simulink model "TelescopeModel"  (R2016a)
settings: Solver=ode45  StartTime=0.0  StopTime=inf  RelTol=1e-3
libraries: simulink x2, vrlib x1
settings Model: Creator=Baris  LastModifiedBy=ds
settings DataIOCC: LimitDataPoints=on  SaveFormat=Array
settings DebuggingCC: SolverPrmCheckMsg=warning  AllowSymbolicDim=off
settings HardwareCC: ProdBitPerPointer=32  ProdLargestAtomicFloat=None  ProdIntDivRoundTo=Undefined  ProdEndianess=Unspecified  ProdWordSize=32  ProdHWDeviceType=32-bit Generic
settings ModelReferenceCC: PropagateSignalLabelsOutOfModel=off
settings ConfigComp: CovModelRefEnable=Off  CovSFcnEnable=off

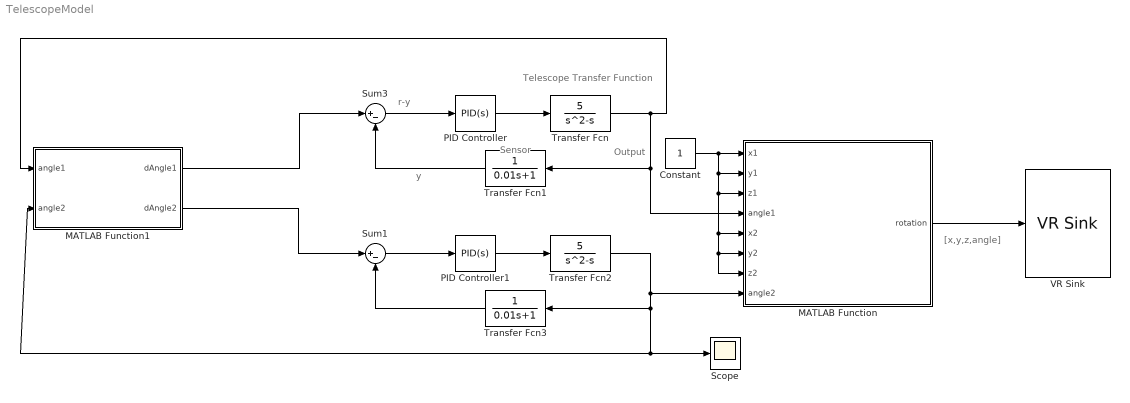
== system TelescopeModel ==
  note: [x,y,z,angle]
  note: r-y
  note: y
  note: Output
  note: Sensor
  note: Telescope Transfer Function
  Constant : Constant
  MATLAB Function : MATLAB Function  TreatAsAtomicUnit=on
  MATLAB Function1 : MATLAB Function  TreatAsAtomicUnit=on
  PID Controller : simulink/Continuous/PID Controller  Controller=PID  TimeDomain=Continuous-time  SampleTime=-1  IntegratorMethod=Forward Euler  FilterMethod=Forward Euler  Form=Ideal  UseFilter=on  ControllerParametersSource=internal  P=9.91044376883815  I=0.179707343353955  D=0.466765758106248  N=123.439816106141  InitialConditionSource=internal  InitialConditionForIntegrator=0  InitialConditionForFilter=0  ExternalReset=none  LimitOutput=off  UpperSaturationLimit=inf  LowerSaturationLimit=-inf  LinearizeAsGain=on  AntiWindupMode=none  Kb=1  TrackingMode=off  Kt=1  PParamMin=[]  PParamMax=[]  IParamMin=[]  IParamMax=[]  DParamMin=[]  DParamMax=[]  NParamMin=[]  NParamMax=[]  KbParamMin=[]  KbParamMax=[]  KtParamMin=[]  KtParamMax=[]  POutMin=[]  POutMax=[]  IOutMin=[]  IOutMax=[]  DOutMin=[]  DOutMax=[]  NOutMin=[]  NOutMax=[]  KbOutMin=[]  KbOutMax=[]  KtOutMin=[]  KtOutMax=[]  IntegratorOutMin=[]  IntegratorOutMax=[]  FilterOutMin=[]  FilterOutMax=[]  SumOutMin=[]  SumOutMax=[]  SumI1OutMin=[]  SumI1OutMax=[]  SumI2OutMin=[]  SumI2OutMax=[]  SumI3OutMin=[]  SumI3OutMax=[]  SumDOutMin=[]  SumDOutMax=[]  SaturationOutMin=[]  SaturationOutMax=[]  IntegratorContinuousStateAttributes=''  IntegratorStateMustResolveToSignalObject=off  IntegratorRTWStateStorageClass=Auto  FilterContinuousStateAttributes=''  FilterStateMustResolveToSignalObject=off  FilterRTWStateStorageClass=Auto  DifferentiatorICPrevScaledInput=0  DifferentiatorOutMin=[]  DifferentiatorOutMax=[]
  PID Controller1 : simulink/Continuous/PID Controller  Controller=PID  TimeDomain=Continuous-time  SampleTime=-1  IntegratorMethod=Forward Euler  FilterMethod=Forward Euler  Form=Ideal  UseFilter=on  ControllerParametersSource=internal  P=9.91044376883815  I=0.179707343353955  D=0.466765758106248  N=123.439816106141  InitialConditionSource=internal  InitialConditionForIntegrator=0  InitialConditionForFilter=0  ExternalReset=none  LimitOutput=off  UpperSaturationLimit=inf  LowerSaturationLimit=-inf  LinearizeAsGain=on  AntiWindupMode=none  Kb=1  TrackingMode=off  Kt=1  PParamMin=[]  PParamMax=[]  IParamMin=[]  IParamMax=[]  DParamMin=[]  DParamMax=[]  NParamMin=[]  NParamMax=[]  KbParamMin=[]  KbParamMax=[]  KtParamMin=[]  KtParamMax=[]  POutMin=[]  POutMax=[]  IOutMin=[]  IOutMax=[]  DOutMin=[]  DOutMax=[]  NOutMin=[]  NOutMax=[]  KbOutMin=[]  KbOutMax=[]  KtOutMin=[]  KtOutMax=[]  IntegratorOutMin=[]  IntegratorOutMax=[]  FilterOutMin=[]  FilterOutMax=[]  SumOutMin=[]  SumOutMax=[]  SumI1OutMin=[]  SumI1OutMax=[]  SumI2OutMin=[]  SumI2OutMax=[]  SumI3OutMin=[]  SumI3OutMax=[]  SumDOutMin=[]  SumDOutMax=[]  SaturationOutMin=[]  SaturationOutMax=[]  IntegratorContinuousStateAttributes=''  IntegratorStateMustResolveToSignalObject=off  IntegratorRTWStateStorageClass=Auto  FilterContinuousStateAttributes=''  FilterStateMustResolveToSignalObject=off  FilterRTWStateStorageClass=Auto  DifferentiatorICPrevScaledInput=0  DifferentiatorOutMin=[]  DifferentiatorOutMax=[]
  Scope : Scope
  Sum1 : Sum  Inputs=|+-
  Sum3 : Sum  Inputs=|+-
  Transfer Fcn : TransferFcn  Numerator=[5]  Denominator=[1 -1 0]
  Transfer Fcn1 : TransferFcn  Denominator=[0.01 1]
  Transfer Fcn2 : TransferFcn  Numerator=[5]  Denominator=[1 -1 0]
  Transfer Fcn3 : TransferFcn  Denominator=[0.01 1]
  VR Sink : vrlib/VR Sink  InstantiateOnLoad=on  SampleTime=0.1  ViewEnable=on  RemoteChange=off  RemoteView=off  FieldsWritten=Scope.rotation.4.1.1.double  WorldFileName=scope123.WRL  AutoView=off  VideoDimensions=[]  AllowVariableSize=off  FigureProperties="{'Position', 'Name', 'Viewpoint', 'CameraBound', 'CameraDirection', 'CameraPosition', 'CameraUpVector', 'ZoomFactor', 'Antialiasing', 'Headlight', 'Lighting', 'NavPanel', 'Sound', 'StatusBar', 'Stereo3D', 'Stereo3DCameraOffset', 'Stereo3DHIT', 'ToolBar', 'Textures', 'Transparency', 'Triad', 'Wireframe', 'NavZones', 'NavMode', 'NavSpeed', 'CaptureFileFormat', 'CaptureFileName', 'Record2DCompressMethod', 'Record2DCompressQuality', 'Record2D', 'Record2DFileName', 'Record2DFPS'; [5.0000000000000000e+00   9.2000000000000000e+01   5.7600000000000000e+02   3.5000000000000000e+02], '', '', 'on', [0.0000000000000000e+00   0.0000000000000000e+00  -1.0000000000000000e+00], [0.0000000000000000e+00   0.0000000000000000e+00   1.0000000000000000e+01], [0.0000000000000000e+00   1.0000000000000000e+00   0.0000000000000000e+00], [1.0000000000000000e+00], 'on', 'on', 'on', 'halfbar', 'on', 'on', 'off', [1.0000000149011612e-01], [0.0000000000000000e+00], 'on', 'on', 'on', 'none', 'off', 'off', 'fly', 'normal', 'tif', '%f_anim_%n.tif', 'auto', [7.5000000000000000e+01], 'off', '%f_anim_%n.avi', 'auto'}"
  wires:
  PID Controller/1 -> Transfer Fcn/1
  Sum3/1 -> PID Controller/1
  Transfer Fcn/1 -> MATLAB Function/4(angle1), Transfer Fcn1/1, MATLAB Function1/1(angle1)
  Transfer Fcn1/1 -> Sum3/2
  PID Controller1/1 -> Transfer Fcn2/1
  Sum1/1 -> PID Controller1/1
  Transfer Fcn2/1 -> MATLAB Function/8(angle2), Scope/1, MATLAB Function1/2(angle2), Transfer Fcn3/1
  Transfer Fcn3/1 -> Sum1/2
  Constant/1 -> MATLAB Function/1(x1), MATLAB Function/7(z2), MATLAB Function/6(y2), MATLAB Function/5(x2), MATLAB Function/3(z1), MATLAB Function/2(y1)
  MATLAB Function/1(rotation) -> VR Sink/1
  MATLAB Function1/1(dAngle1) -> Sum3/1
  MATLAB Function1/2(dAngle2) -> Sum1/1

== matlab function TelescopeModel/MATLAB Function1 ==
  data: angle1 input; dAngle1 output; angle2 input; dAngle2 output
function [dAngle1,dAngle2] = fcn(angle1, angle2)
    % initialize values if they haven't been set
    dAngle1 = 0;
    dAngle2 = 0;
    currentState = load('stardata.mat');
    stars = currentState.stars;
    persistent desiredAngle1;
    persistent desiredAngle2;
    persistent currentStarIndex;
    if isempty(desiredAngle1)
        currentStarIndex = 1;
        desiredAngle1 = stars(1,1);
        desiredAngle2 = stars(1,2);
        dAngle1 = desiredAngle1;
        dAngle2 = desiredAngle2;
    end
    % change desired angle once reached and two photos have been taken
    if angle1 > desiredAngle1-0.01 && angle1< desiredAngle1+0.01 && angle2 > desiredAngle2-0.01 && angle2 < desiredAngle2+0.01
        %pause(10); %must be a better way to do this than literally pausing
        %the program for ten seconds at a time
        if currentStarIndex ~= 100
            currentStarIndex = currentStarIndex + 1;
            desiredAngle1 = stars(currentStarIndex,1);
            desiredAngle2 = stars(currentStarIndex,2);
            dAngle1 = desiredAngle1;
            dAngle2 = desiredAngle2;
        else
            disp('all over');
        end
    else
        dAngle1 = desiredAngle1;
        dAngle2 = desiredAngle2;
    end
end

== matlab function TelescopeModel/MATLAB Function ==
  data: x1 input; rotation output; y1 input; z1 input; angle1 input; x2 input; y2 input; z2 input; angle2 input
function rotation = fcn(x1, y1, z1, angle1, x2, y2, z2, angle2)

if((x1*x1 + y1*y1 + z1*z1) ~= 1)
    NormeCarree = (x1*x1 + y1*y1 + z1*z1);
    invNorme = (1/sqrt(NormeCarree));
    x1 = x1 * invNorme;
    y1 = y1 * invNorme;
    z1 = z1 * invNorme;
end

if((x2*x2 + y2*y2 + z2*z2) ~= 1)
    NormeCarree = (x2*x2 + y2*y2 + z2*z2);
    invNorme = (1/sqrt(NormeCarree));
    x2 = x2 * invNorme;
    y2 = y2 * invNorme;
    z2 = z2 * invNorme;
end

% convert axis-angle 1 to quaternion
w1 = cos(angle1/2);
s = sin(angle1/2);
x1 = x1 * s;
y1 = y1 * s;
z1 = z1 * s;

% convert axis-angle 2 to quaternion
w2 = cos(angle2/2);
s = sin(angle2/2);
x2 = x2 * s;
y2 = y2 * s;
z2 = z2 * s;

angleFinal = w2*w1 - x2*x1 - y2*y1 - z2*z1;
xFinal = x2*w1 + w2*x1 + y2*z1 - z2*y1;
yFinal = w2*y1 - x2*z1 + y2*w1 + z2*x1;
zFinal = w2*z1 + x2*y1 - y2*x1 + z2*w1;

% now extract the result
if(angleFinal == 1 || angleFinal == -1)
    angleFinal = 0;
    xFinal = 1; yFinal = 0; zFinal = 0;
else
    s = sqrt(1-angleFinal*angleFinal);
    angleFinal = 2 * acos(angleFinal);
    
    if (abs(s) < 0.001) s = 1;
        xFinal = xFinal / s;
        yFinal = yFinal / s;
        zFinal = zFinal / s;
    end
end
rotation = zeros(1,4);
rotation = [xFinal yFinal zFinal angleFinal];
end
